simulink model "VerificaHinf"  (R2025b)
settings: Solver=ode4  StartTime=0.0  StopTime=10.0  FixedStep=0.001  RelTol=1e-3
undefined symbols (not defined in the file): A, B, C, C_EIG, D, x0_EIG
libraries: cstblocks x1
settings Model: Creator=salvo  LastModifiedBy=salvo

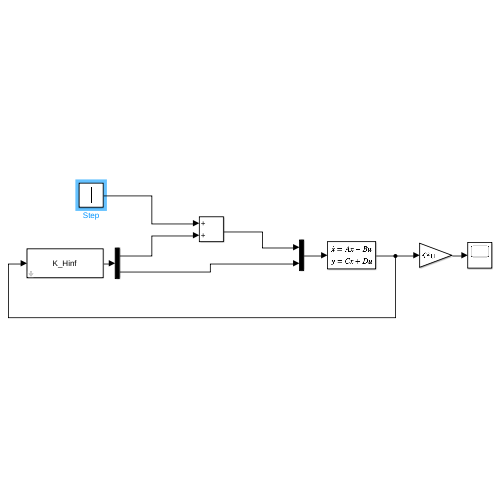
[thumbnail: Simulink's stored preview of the top-level diagram]
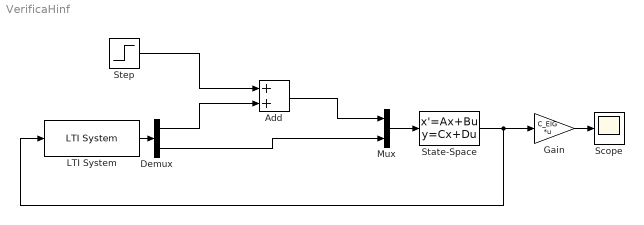
== system VerificaHinf ==
  Add : Sum
  Demux : Demux  Outputs=2
  Gain : Gain  Gain=C_EIG  Multiplication=Matrix(K*u)
  LTI System : cstblocks/LTI System  sys=K_Hinf  IC=[]  PadeOrder=0
  Mux : Mux  Inputs=2
  Scope : Scope
      settings: ActiveDisplayYMinimum=-87.441683152749519  ActiveDisplayYMaximum=139.11881597487454
  State-Space : StateSpace  A=A  B=B  C=C  D=D  InitialCondition=x0_EIG
  Step : Step  Before=500  After=100  SampleTime=0
  wires:
  State-Space/1 -> LTI System/1, Gain/1
  Gain/1 -> Scope/1
  Step/1 -> Add/1
  Mux/1 -> State-Space/1
  LTI System/1 -> Demux/1
  Add/1 -> Mux/1
  Demux/1 -> Add/2
  Demux/2 -> Mux/2
